simulink model "Sun_Mission"  (R2021a)
settings: Solver=VariableStepAuto  StartTime=0.0  StopTime=200  RelTol=1e-3
values from neighbouring files (symbols this model uses):
  dtheta_LMO = sqrt(muy/r_LMO^3)    [Parameters.m]    (also in Spacecraft_Attitude_States.m)
  I = [10 0 0;0 5 0;0 0 7.5]    [Parameters.m]    (also in Spacecraft_Attitude_States.m)
  i0_LMO = pi/6    (= 0.523598775598)    [Parameters.m]    (also in Spacecraft_Attitude_States.m)
  K = 5    [Parameters.m]    (also in Spacecraft_Attitude_States.m)
  Omega0_LMO = pi/9    (= 0.349065850399)    [Parameters.m]    (also in Spacecraft_Attitude_States.m)
  P = 10*eye(3)    [Parameters.m]    (also in Spacecraft_Attitude_States.m)
  theta0_LMO = pi/3    (= 1.0471975512)    [Parameters.m]    (also in Spacecraft_Attitude_States.m)
settings Model: Creator=VTX  LastModifiedBy=VTX

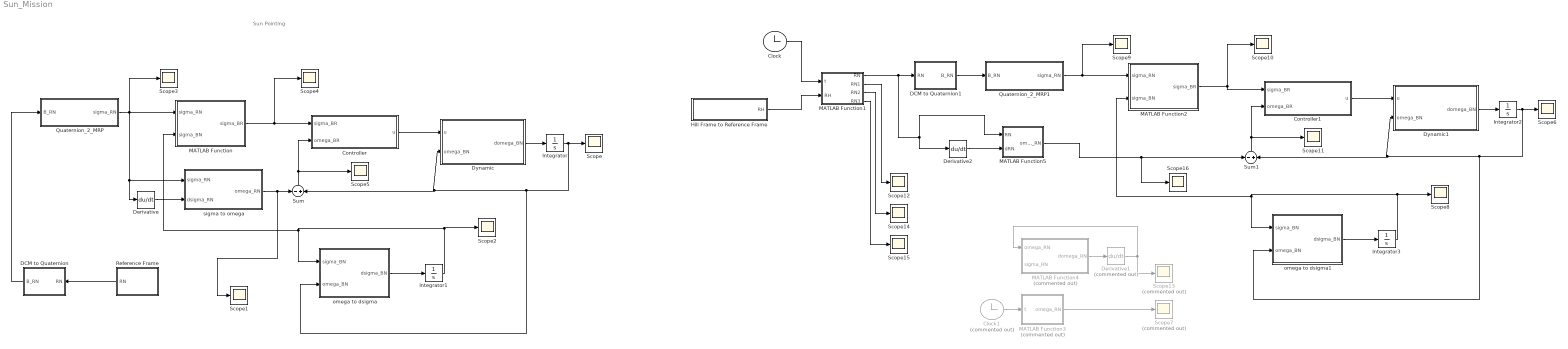
== system Sun_Mission ==
  note: Sun Pointing
  Clock : Clock
  Clock1 : Clock  Commented=on
  Controller : MATLAB Function  TreatAsAtomicUnit=on
  Controller1 : MATLAB Function  TreatAsAtomicUnit=on
  DCM to Quaternion : MATLAB Function  TreatAsAtomicUnit=on
  DCM to Quaternion1 : MATLAB Function  TreatAsAtomicUnit=on
  Derivative : Derivative
  Derivative1 : Derivative  Commented=on
  Derivative2 : Derivative
  Dynamic : MATLAB Function  TreatAsAtomicUnit=on
  Dynamic1 : MATLAB Function  TreatAsAtomicUnit=on
  Hill Frame to Reference Frame : MATLAB Function  TreatAsAtomicUnit=on
  Integrator : Integrator  InitialCondition=[1;1.75;-2.2]*pi/180
  Integrator1 : Integrator  InitialCondition=[0.3;-0.4;0.5]
  Integrator2 : Integrator  InitialCondition=[1;1.75;-2.2]*pi/180
  Integrator3 : Integrator  InitialCondition=[0.3;-0.4;0.5]
  MATLAB Function : MATLAB Function  TreatAsAtomicUnit=on
  MATLAB Function1 : MATLAB Function  TreatAsAtomicUnit=on
  MATLAB Function2 : MATLAB Function  TreatAsAtomicUnit=on
  MATLAB Function3 : MATLAB Function  Commented=on  TreatAsAtomicUnit=on
  MATLAB Function4 : MATLAB Function  Commented=on  TreatAsAtomicUnit=on
  MATLAB Function5 : MATLAB Function  TreatAsAtomicUnit=on
  Quaternion_2_MRP : MATLAB Function  TreatAsAtomicUnit=on
  Quaternion_2_MRP1 : MATLAB Function  TreatAsAtomicUnit=on
  Reference Frame : MATLAB Function  TreatAsAtomicUnit=on
  Scope{,1..6,8..12,14..16} (15 alike) : Scope
  Scope13 : Scope  Commented=on
  Scope7 : Scope  Commented=on
  Sum : Sum  Inputs=-|+
  Sum1 : Sum  Inputs=-|+
  omega to dsigma : MATLAB Function  TreatAsAtomicUnit=on
  omega to dsigma1 : MATLAB Function  TreatAsAtomicUnit=on
  sigma to omega : MATLAB Function  TreatAsAtomicUnit=on
  wires:
  Dynamic/1(domega_BN) -> Integrator/1
  Integrator/1 -> Scope/1, omega to dsigma/2(omega_BN), Sum/2, Dynamic/2(omega_BN)
  Controller/1(u) -> Dynamic/1(u)
  Reference Frame/1(RN) -> DCM to Quaternion/1(RN)
  omega to dsigma/1(dsigma_BN) -> Integrator1/1
  Integrator1/1 -> Scope2/1, MATLAB Function/2(sigma_BN), omega to dsigma/1(sigma_BN)
  DCM to Quaternion/1(B_RN) -> Quaternion_2_MRP/1(B_RN)
  MATLAB Function/1(sigma_BR) -> Scope4/1, Controller/1(sigma_BR)
  Sum/1 -> Scope5/1, Controller/2(omega_BR)
  sigma to omega/1(omega_RN) -> Scope1/1, Sum/1
  Derivative/1 -> sigma to omega/2(dsigma_RN)
  Quaternion_2_MRP/1(sigma_RN) -> Derivative/1, sigma to omega/1(sigma_RN), Scope3/1, MATLAB Function/1(sigma_RN)
  Hill Frame to Reference Frame/1(RH) -> MATLAB Function1/2(RH)
  Clock/1 -> MATLAB Function1/1(t)
  Integrator3/1 -> Scope8/1, MATLAB Function2/2(sigma_BN), omega to dsigma1/1(sigma_BN)
  MATLAB Function3/1(omega_RN) -> Scope7/1
  MATLAB Function2/1(sigma_BR) -> Controller1/1(sigma_BR), Scope10/1
  omega to dsigma1/1(dsigma_BN) -> Integrator3/1
  Integrator2/1 -> Scope6/1, omega to dsigma1/2(omega_BN), Sum1/2, Dynamic1/2(omega_BN)
  Controller1/1(u) -> Dynamic1/1(u)
  Dynamic1/1(domega_BN) -> Integrator2/1
  Sum1/1 -> Scope11/1, Controller1/2(omega_BR)
  DCM to Quaternion1/1(B_RN) -> Quaternion_2_MRP1/1(B_RN)
  Clock1/1 -> MATLAB Function3/1(t)
  Quaternion_2_MRP1/1(sigma_RN) -> MATLAB Function2/1(sigma_RN), Scope9/1
  MATLAB Function1/1(RN) -> MATLAB Function5/1(RN), Derivative2/1, DCM to Quaternion1/1(RN)
  MATLAB Function1/2(RN1) -> Scope12/1
  MATLAB Function1/3(RN2) -> Scope14/1
  MATLAB Function1/4(RN3) -> Scope15/1
  MATLAB Function4/1(domega_RN) -> Derivative1/1
  Derivative1/1 -> MATLAB Function4/1(omega_RN), Scope13/1
  Derivative2/1 -> MATLAB Function5/2(dRN)
  MATLAB Function5/1(omega_RN) -> Scope16/1, Sum1/1

== matlab function Sun_Mission/Controller1 ==
  data: sigma_BR input; u output; omega_BR input; K parameter; P parameter
function u = fcn(sigma_BR,omega_BR,K,P)

    u = -K*sigma_BR - P*omega_BR;
end

== matlab function Sun_Mission/MATLAB Function3 ==
  data: omega_RN output; i0_LMO parameter; theta0_LMO parameter; dtheta_LMO parameter; t input
function omega_RN = fcn(i0_LMO,theta0_LMO,dtheta_LMO,t)
    omega_RN = [(sin(theta0_LMO + dtheta_LMO*t)*sin(i0_LMO)) cos(theta0_LMO + dtheta_LMO*t) 0; ...
             (cos(theta0_LMO + dtheta_LMO*t)*sin(i0_LMO)) -sin(theta0_LMO + dtheta_LMO*t) 0; ...
             cos(i0_LMO) 0 1]*[0 0 dtheta_LMO]';    
end

== matlab function Sun_Mission/Dynamic1 ==
  data: u input; domega_BN output size=3; omega_BN input; I parameter
function domega_BN = fcn(u,omega_BN, I)
    domega_BN = inv(I)*(cross(omega_BN,(I*omega_BN)) + u);
end

== matlab function Sun_Mission/MATLAB Function2 ==
  data: sigma_BR output; sigma_RN input; sigma_BN input
function sigma_BR = fcn(sigma_RN, sigma_BN)
    sigma_BR = ((1 - norm(sigma_RN)^2)*sigma_BN - (1 - norm(sigma_BN)^2)*sigma_RN + 2*cross(sigma_BN,sigma_RN))/(1 + norm(sigma_RN)^2*norm(sigma_BN)^2 + 2*dot(sigma_RN,sigma_BN));
end

== matlab function Sun_Mission/Quaternion_2_MRP1 ==
  data: B_RN input; sigma_RN output
function sigma_RN  = fcn(B_RN)
    sigma1 = B_RN(2)/(1 + B_RN(1));
    sigma2 = B_RN(3)/(1 + B_RN(1));
    sigma3 = B_RN(4)/(1 + B_RN(1));
    
    sigma_RN = [sigma1 sigma2 sigma3]';

    if norm(sigma_RN) >= 1
        sigma1 = -B_RN(2)/(1 - B_RN(1));
        sigma2 = -B_RN(3)/(1 - B_RN(1));
        sigma3 = -B_RN(4)/(1 - B_RN(1));
    
        sigma_RN = [sigma1 sigma2 sigma3]';
    end   
end

== matlab function Sun_Mission/Controller ==
  data: sigma_BR input; u output; omega_BR input; K parameter; P parameter
function u = fcn(sigma_BR,omega_BR,K,P)

    u = -K*sigma_BR - P*omega_BR;
end

== matlab function Sun_Mission/MATLAB Function4 ==
  data: domega_RN output size=3; omega_RN input; sigma_RN input; I parameter; K parameter; P parameter
function domega_RN = fcn(omega_RN,sigma_RN, I,K, P)
    % domega_RN = inv(I)*(-cross(omega_RN,(I*omega_RN)));
    domega_RN = inv(I)*(-P*omega_RN - K*sigma_RN);
end

== matlab function Sun_Mission/omega to dsigma1 ==
  data: sigma_BN input; dsigma_BN output; omega_BN input
function dsigma_BN = fcn(sigma_BN,omega_BN)
   sigma_tilde = [0 -sigma_BN(3) sigma_BN(2);sigma_BN(3) 0 -sigma_BN(1);-sigma_BN(2) sigma_BN(1) 0];
   dsigma_BN = 1/4*((1 - dot(sigma_BN,sigma_BN))*eye(3) + 2*sigma_tilde + 2*sigma_BN*sigma_BN')*omega_BN;
end

== matlab function Sun_Mission/MATLAB Function5 ==
  data: RN input; omega_RN output; dRN input
function omega_RN = fcn(RN,dRN)
    omega_RN_tidle = -dRN*RN';
    o1 = omega_RN_tidle(3,2);
    o2 = omega_RN_tidle(1,3);
    o3 = omega_RN_tidle(2,1);
    omega_RN = [o1 o2 o3]';
end

== matlab function Sun_Mission/Dynamic ==
  data: u input; domega_BN output size=3; omega_BN input; I parameter
function domega_BN = fcn(u,omega_BN, I)
    domega_BN = inv(I)*(cross(omega_BN,(I*omega_BN)) + u);
end

== matlab function Sun_Mission/DCM to Quaternion ==
  data: RN input; B_RN output size=4
function B_RN = fcn(RN)
    trace = RN(1,1) + RN(2,2) + RN(3,3);
    beta0 = (0.25*(1 + trace));
    beta1 = (0.25*(1 + 2*RN(1,1) - trace));
    beta2 = (0.25*(1 + 2*RN(2,2) - trace));
    beta3 = (0.25*(1 + 2*RN(3,3) - trace));
    
    m = max([beta0 beta1 beta2 beta3]);

    B0 = 0; B1 = 0; B2 = 0; B3 = 0;
    
    if beta0 == m
        B0 = sqrt(beta0);
        B1 = (RN(2,3)-RN(3,2))/(4*B0);
        B2 = (RN(3,1)-RN(1,3))/(4*B0);
        B3 = (RN(1,2)-RN(2,1))/(4*B0);
    elseif beta1 == m
        B1 = sqrt(beta1);
        B0 = (RN(2,3)-RN(3,2))/(4*B1);
        B2 = (RN(1,2)+RN(2,1))/(4*B1);
        B3 = (RN(3,1)+RN(1,3))/(4*B1);
    elseif beta2 == m
        B2 = sqrt(beta2);
        B0 = (RN(3,1)-RN(1,3))/(4*B2);
        B1 = (RN(1,2)+RN(2,1))/(4*B2);
        B3 = (RN(2,3)+RN(3,2))/(4*B2);
    elseif beta3 == m
        B3 = sqrt(beta3);
        B0 = (RN(1,2)-RN(2,1))/(4*B3);
        B1 = (RN(3,1)+RN(1,3))/(4*B3);
        B2 = (RN(2,3)+RN(3,2))/(4*B3);
    end
    
    B_RN = [B0 B1 B2 B3]';
end

== matlab function Sun_Mission/Quaternion_2_MRP ==
  data: B_RN input; sigma_RN output
function sigma_RN = fcn(B_RN)
    sigma1 = B_RN(2)/(1 + B_RN(1));
    sigma2 = B_RN(3)/(1 + B_RN(1));
    sigma3 = B_RN(4)/(1 + B_RN(1));
    
    sigma_RN = [sigma1 sigma2 sigma3]';
    if norm(sigma_RN) >= 1
       sigma_RN = -sigma_RN; 
    end
end

== matlab function Sun_Mission/Reference Frame ==
  data: RN output
function RN = fcn()
    RN = [-1 0 0;0 0 1;0 1 0];
end

== matlab function Sun_Mission/omega to dsigma ==
  data: sigma_BN input; dsigma_BN output; omega_BN input
function dsigma_BN = fcn(sigma_BN,omega_BN)
   sigma_tilde = [0 -sigma_BN(3) sigma_BN(2);sigma_BN(3) 0 -sigma_BN(1);-sigma_BN(2) sigma_BN(1) 0];
   dsigma_BN = 1/4*((1 - dot(sigma_BN,sigma_BN))*eye(3) + 2*sigma_tilde + 2*sigma_BN*sigma_BN')*omega_BN;
end

== matlab function Sun_Mission/MATLAB Function ==
  data: sigma_BR output; sigma_RN input; sigma_BN input
function sigma_BR = fcn(sigma_RN, sigma_BN)
    sigma_BR = ((1 - norm(sigma_RN)^2)*sigma_BN - (1 - norm(sigma_BN)^2)*sigma_RN + 2*cross(sigma_BN,sigma_RN))/(1 + norm(sigma_RN)^2*norm(sigma_BN)^2 + 2*dot(sigma_RN,sigma_BN));
end

== matlab function Sun_Mission/sigma to omega ==
  data: sigma_RN input; omega_RN output; dsigma_RN input
function omega_RN = fcn(sigma_RN,dsigma_RN)
    sigma_tilde = [0 -sigma_RN(3) sigma_RN(2);sigma_RN(3) 0 -sigma_RN(1);-sigma_RN(2) sigma_RN(1) 0];
    omega_RN = 4/(1 + dot(sigma_RN,sigma_RN))^2*((1 - dot(sigma_RN,sigma_RN))*eye(3) - 2*sigma_tilde + 2*sigma_RN*sigma_RN')*dsigma_RN;
end

== matlab function Sun_Mission/Hill Frame to Reference Frame ==
  data: RH output
function RH = fcn()
RH = [-1 0 0;0 1 0;0 0 -1];
end

== matlab function Sun_Mission/MATLAB Function1 ==
  data: RN output; t input; RH input; Omega0_LMO parameter; i0_LMO parameter; theta0_LMO parameter; dtheta_LMO parameter; RN1 output; RN2 output; RN3 output
function [RN,RN1,RN2,RN3] = fcn(t, RH,Omega0_LMO, i0_LMO, theta0_LMO, dtheta_LMO)
    %% Rotate about z axis
    Cz1 = [cos(Omega0_LMO) sin(Omega0_LMO) 0;-sin(Omega0_LMO) cos(Omega0_LMO) 0;0 0 1];

    %% Rotate about x axis
    Cx2 = [1 0 0;0 cos(i0_LMO) sin(i0_LMO);0 -sin(i0_LMO) cos(i0_LMO)];
    
    %% Rotate about z axis
    Cz3 = [cos(theta0_LMO + dtheta_LMO*t) sin(theta0_LMO + dtheta_LMO*t) 0;-sin(theta0_LMO + dtheta_LMO*t) cos(theta0_LMO + dtheta_LMO*t) 0;0 0 1];

    %% DCM from Inertial Frame to Hill Frame
    HN = Cz3*Cx2*Cz1;
    
    %% DCm from Inertial Frame to Reference Frame
    RN = RH*HN;
    RN1 = RN(:,1);
    RN2 = RN(:,2);
    RN3 = RN(:,3);
end

== matlab function Sun_Mission/DCM to Quaternion1 ==
  data: RN input; B_RN output size=4
function B_RN = fcn(RN)
    trace = RN(1,1) + RN(2,2) + RN(3,3);
    beta0 = (0.25*(1 + trace));
    beta1 = (0.25*(1 + 2*RN(1,1) - trace));
    beta2 = (0.25*(1 + 2*RN(2,2) - trace));
    beta3 = (0.25*(1 + 2*RN(3,3) - trace));
    
    m = max([beta0 beta1 beta2 beta3]);

    B0 = 0; B1 = 0; B2 = 0; B3 = 0;
    
    if beta0 == m
        B0 = sqrt(beta0);
        B1 = (RN(2,3)-RN(3,2))/(4*B0);
        B2 = (RN(3,1)-RN(1,3))/(4*B0);
        B3 = (RN(1,2)-RN(2,1))/(4*B0);
    elseif beta1 == m
        B1 = sqrt(beta1);
        B0 = (RN(2,3)-RN(3,2))/(4*B1);
        B2 = (RN(1,2)+RN(2,1))/(4*B1);
        B3 = (RN(3,1)+RN(1,3))/(4*B1);
    elseif beta2 == m
        B2 = sqrt(beta2);
        B0 = (RN(3,1)-RN(1,3))/(4*B2);
        B1 = (RN(1,2)+RN(2,1))/(4*B2);
        B3 = (RN(2,3)+RN(3,2))/(4*B2);
    elseif beta3 == m
        B3 = sqrt(beta3);
        B0 = (RN(1,2)-RN(2,1))/(4*B3);
        B1 = (RN(3,1)+RN(1,3))/(4*B3);
        B2 = (RN(2,3)+RN(3,2))/(4*B3);
    end
    
    B_RN = [B0 B1 B2 B3]';
end
